simulink model "AFDNFSmodelSPA"  (R2017b)
settings: Solver=ode45  StartTime=0.0  StopTime=1400  FixedStep=1e-3  RelTol=1e-8  EnableMultiTasking=on
PostLoadFcn:
  | run('Methods/NFSOnLoad');
InitFcn:
  | run('Methods/AFDSimInit')
StopFcn:
  | run('Methods/NFSOnLoad');
values from neighbouring files (symbols this model uses):
  nfs = TransferFunction('Plot','true')    [Main.m]    (also in NFSDatabase.sldd = SI
                Imperial
                28184.4409185639)
undefined symbols (not defined in the file or in its folder): Continuous, desired, Earth, F, K_lat, K_long, Kobsvlat, Kobsvlong, lat, latsys, Light, long, longsys, MIL, Newton, Raphson, sigbuilder_block, Time, WGS84
libraries: simulink x6, aerolibtransform2 x2, aerolibwind2 x2, ModelsLibrary x1, ctrlSharedLib x1, sharedutil x1
(part 1 of 4)
settings Model: Creator=AHKh PC  LastModifiedBy=AHKh
settings SolverCC: ZeroCrossAlgorithm=Adaptive  AutoInsertRateTranBlk=on
settings DataIOCC: SaveFormat=Array  SignalLoggingSaveFormat=ModelDataLogs  SaveOutput=off
settings OptimizationCC: ExpressionDepthLimit=2147483647  LifeSpan=inf
settings DebuggingCC: UnderspecifiedInitializationDetection=Classic  MergeDetectMultiDrivingBlocksExec=none  SolverPrmCheckMsg=warning  FcnCallInpInsideContextMsg=warning  StateNameClashWarn=warning  SFUnexpectedBacktrackingDiag=warning  SFNoUnconditionalDefaultTransitionDiag=warning  SFExecutionAtInitializationDiag=none
settings HardwareCC: ProdBitPerPointer=32  ProdBitPerSizeT=32  ProdBitPerPtrDiffT=32  ProdLargestAtomicFloat=None  ProdIntDivRoundTo=Undefined  ProdEndianess=Unspecified  ProdWordSize=32  ProdHWDeviceType=32-bit Generic
settings ModelReferenceCC: PropagateSignalLabelsOutOfModel=off
settings CodeAppCC: StateflowObjectComments=on
settings GRTTargetCC: TargetLangStandard=C89/C90 (ANSI)  GeneratePreprocessorConditionals=Disable all
settings ConfigComp: CovMetricSettings=dw  CovHtmlReporting=on  CovSaveCumulativeToWorkspaceVar=on  CovSaveSingleToWorkspaceVar=on  CovExternalEMLEnable=off

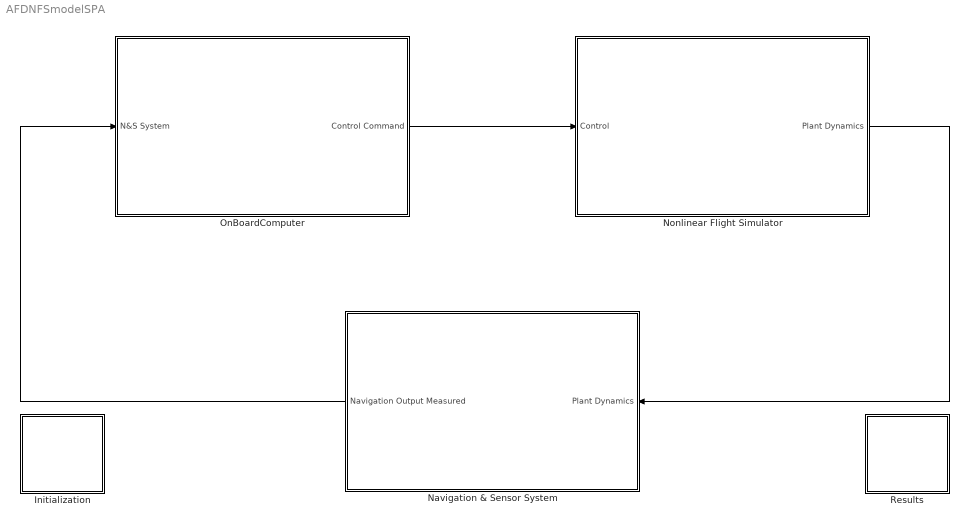
== system AFDNFSmodelSPA ==
  Initialization : Subsystem
      settings: OpenFcn=|
      | % edit('Methods/AFDSimInit.m')
      | !NFSData/NFS Data.xlsx
      mask Display: image(imread('iData/Initialization'))
  Navigation & Sensor System : Subsystem
      mask Display: image(imread('iData/NavigationSystem'))
  Nonlinear Flight Simulator : Subsystem
      mask Display: image(imread('iData/LockheedMartinVARIOUS'));
  OnBoardComputer : Subsystem
      mask Display: image(imread('iData/OnBoardComputerESAPathfinder'));
  Results : Subsystem
      settings: OpenFcn=|
      | cd 'Methods';
      | Plotter(ned_position,euler_angles,control_commands,tout)
      | cd ..
      mask Display: image(imread('iData/Initialization'))
  wires:
  OnBoardComputer/1(Control Command) -> Nonlinear Flight Simulator/1(Control)
  Navigation & Sensor System/1(Navigation Output Measured) -> OnBoardComputer/1(N&S System)
  Nonlinear Flight Simulator/1(Plant Dynamics) -> Navigation & Sensor System/1(Plant Dynamics)

== system AFDNFSmodelSPA/Initialization ==

== system AFDNFSmodelSPA/Navigation & Sensor System ==
  note: Major Contributions
      | 1- Pitotube Model Shall be added
      | 2- GPS Model shall be added
      | 3-
      | 4-
  note: 0-Ideal Measurement - full-state feedback
      |
      | 1- Test Model - no filter propagation - model based propagation
      |
      | 2- Pure noise added to all measurements - no filter - full-state feedback
      |
      | 3- Pure noise added to all measurements - Linear Kalman Filter - gyro and accelerometer feedback - postion ideal
      |
      | 4- Pure noise added to all measurements - Extended Kalman Filter - gyro and accelerometer feedback - postion ideal
      |
      | 5- Pure noise added to all measurements - Unscented Kalman Filter - gyro and accelerometer feedback - postion ideal
      |
      | 6 - Comprehensive model of Gyro and Accelerometer - Extended Kalman Filter - Ideal Position
      |
      | 7 - Comprehensive model of Gyro and Accelerometer - Unscented Kalman Filter - Ideal Position
      |
      | 8 - Adding GPS to equations
  Plant Dynamics : Inport
  Navigation Model : Subsystem  Variant=on
  Navigation Output Measured : Outport
  wires:
  Plant Dynamics/1 -> Navigation Model/1(In)
  Navigation Model/1(Out) -> Navigation Output Measured/1

== system AFDNFSmodelSPA/Nonlinear Flight Simulator ==
  Control : Inport
  6DoF Nonlinear Flight Equations of Motion (Rigid Body) : Subsystem
  Bus Creator : BusCreator  Inputs=7
  Forces and Moments : Subsystem
  Ground1 : Ground
  Initialization : Subsystem
  Plot : Subsystem
  Scope : Scope
  Scope1 : Scope
  Scope4 : Scope
  Plant Dynamics : Outport
  wires:
  Forces and Moments/1(Force (Body)) -> Scope1/1, 6DoF Nonlinear Flight Equations of Motion (Rigid Body)/1(Forces (F) (Body))
  Forces and Moments/2(Moment (Body)) -> Scope4/1, 6DoF Nonlinear Flight Equations of Motion (Rigid Body)/2(Moments (M) (Body))
  6DoF Nonlinear Flight Equations of Motion (Rigid Body)/1(Linear Velocity (Body)) -> Forces and Moments/1(Linear Velocity), Bus Creator/1, Plot/1(Linear Velocity (Body))  "Linear Velocity"
  Initialization/3(Initial Inertia tensor) -> 6DoF Nonlinear Flight Equations of Motion (Rigid Body)/5(Inertia Tensor (I))
  Initialization/4(Inertia tensor Change Rate) -> 6DoF Nonlinear Flight Equations of Motion (Rigid Body)/6(Inertia Tensor Change Rate (Idot))
  Control/1 -> Forces and Moments/3(Control)
  Initialization/2(Mass Consumption Rate) -> 6DoF Nonlinear Flight Equations of Motion (Rigid Body)/4(Mass Consumption Rate)
  Initialization/1(Initial Mass) -> 6DoF Nonlinear Flight Equations of Motion (Rigid Body)/3(Initial Mass)
  Initialization/5(Initial Linear Velocity Vector) -> 6DoF Nonlinear Flight Equations of Motion (Rigid Body)/7(Initial Linear Velocity Vector)
  Initialization/6(Initial Angular Velocity Vector) -> 6DoF Nonlinear Flight Equations of Motion (Rigid Body)/8(Initial Angular Velocity Vector)
  Initialization/7(Initial Euler Angles) -> 6DoF Nonlinear Flight Equations of Motion (Rigid Body)/9(Initial Euler Angles)
  6DoF Nonlinear Flight Equations of Motion (Rigid Body)/2(Angular Velocity (Body)) -> Forces and Moments/2(Angular Velocity), Bus Creator/2, Plot/2(Angular Velocity (Body))  "Angular Velocity"
  6DoF Nonlinear Flight Equations of Motion (Rigid Body)/4(Angular Acceleration (Body)) -> Bus Creator/4, Plot/4(Angular Acceleration (Body))  "Angular Acceleration"
  Initialization/8(Initial Location (NED)) -> 6DoF Nonlinear Flight Equations of Motion (Rigid Body)/10(Initial Location (NED))
  6DoF Nonlinear Flight Equations of Motion (Rigid Body)/3(Linear Acceleration (Body)) -> Bus Creator/3, Plot/3(Linear Acceleration (Body))  "Linear Acceleration"
  6DoF Nonlinear Flight Equations of Motion (Rigid Body)/7(Velocity (NED)) -> Bus Creator/7, Plot/7(Velocity (NED))  "Velocity"
  Ground1/1 -> Scope/1
  6DoF Nonlinear Flight Equations of Motion (Rigid Body)/6(Position (NED)) -> Forces and Moments/5(Position), Bus Creator/6, Plot/6(Position (NED))  "Position"
  6DoF Nonlinear Flight Equations of Motion (Rigid Body)/5(Euler Angles) -> Forces and Moments/4(Attitute), Bus Creator/5, Plot/5(Euler Angles)  "Euler Angles"
  Bus Creator/1 -> Plant Dynamics/1
  6DoF Nonlinear Flight Equations of Motion (Rigid Body)/8(T_BI) -> Forces and Moments/6(T_BI)

== system AFDNFSmodelSPA/OnBoardComputer ==
  N&S System : Inport
  Control System : Subsystem
  Guidance Algorithm : Subsystem
  Control Command : Outport
  wires:
  N&S System/1 -> Control System/2(N&S System), Guidance Algorithm/1(N&S System)
  Guidance Algorithm/1(Guidance Command) -> Control System/1(Guidance)
  Control System/1(Control Command) -> Control Command/1

== system AFDNFSmodelSPA/Results ==

== system AFDNFSmodelSPA/Navigation & Sensor System/Navigation Model ==
  In : Inport
  00-Ideal Measurement : Subsystem  VariantControl=NavigationSelector == 0
  01-Test Model : Subsystem  VariantControl=NavigationSelector == 1
  02-Pure Noise Full-State Feedback : Subsystem  VariantControl=NavigationSelector == 2
  03-Pure Noise Linear Kalman Filter (LKF) : Subsystem  VariantControl=NavigationSelector == 3
  Out : Outport

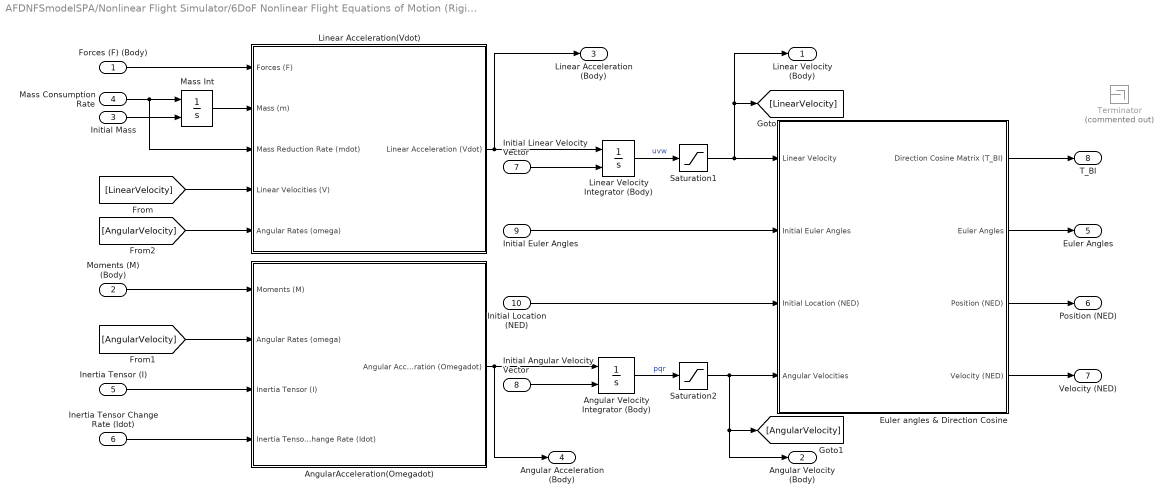
== system AFDNFSmodelSPA/Nonlinear Flight Simulator/6DoF Nonlinear Flight Equations of Motion (Rigid Body) ==
  Forces (F) (Body) : Inport
  Moments (M) (Body) : Inport  Port=2  PortDimensions=[3,1]
  Initial Mass : Inport  Port=3
  Mass Consumption Rate : Inport  Port=4
  Inertia Tensor (I) : Inport  Port=5
  Inertia Tensor Change Rate (Idot) : Inport  Port=6
  Initial Linear Velocity Vector : Inport  Port=7
  Initial Angular Velocity Vector : Inport  Port=8
  Initial Euler Angles : Inport  Port=9
  Initial Location (NED) : Inport  Port=10
  Angular Velocity Integrator (Body) : Integrator  InitialConditionSource=external  InitialCondition=nfs.angularvel0
  AngularAcceleration(Omegadot) : Subsystem
  Euler angles & Direction Cosine : Subsystem
  Linear Acceleration(Vdot) : Subsystem
  Linear Velocity Integrator (Body) : Integrator  InitialConditionSource=external  InitialCondition=nfs.crusevelvec  ContinuousStateAttributes='BodyVelocity'
  Mass Int : Integrator  InitialConditionSource=external  InitialCondition=nfs.crusevelvec  ContinuousStateAttributes='BodyVelocity'
  Saturation1 : Saturate  UpperLimit=500  LowerLimit=-500
  Saturation2 : Saturate  UpperLimit=500  LowerLimit=-500
  Terminator : Terminator  Commented=on
  Linear Velocity (Body) : Outport
  Angular Velocity (Body) : Outport  Port=2
  Linear Acceleration (Body) : Outport  Port=3
  Angular Acceleration (Body) : Outport  Port=4
  Euler Angles : Outport  Port=5
  Position (NED) : Outport  Port=6
  Velocity (NED) : Outport  Port=7
  T_BI : Outport  Port=8
  wires:
  Initial Mass/1 -> Mass Int/2
  Mass Int/1 -> Linear Acceleration(Vdot)/2(Mass (m))
  Mass Consumption Rate/1 -> Linear Acceleration(Vdot)/3(Mass Reduction Rate (mdot)), Mass Int/1
  Linear Velocity Integrator (Body)/1 -> Saturation1/1  "uvw"
  Angular Velocity Integrator (Body)/1 -> Saturation2/1  "pqr"
  Inertia Tensor (I)/1 -> AngularAcceleration(Omegadot)/3(Inertia Tensor (I))
  Inertia Tensor Change Rate (Idot)/1 -> AngularAcceleration(Omegadot)/4(Inertia Tensor Change Rate (Idot))
  Euler angles & Direction Cosine/1(Direction Cosine Matrix (T_BI)) -> T_BI/1
  Initial Location (NED)/1 -> Euler angles & Direction Cosine/3(Initial Location (NED))
  Forces (F) (Body)/1 -> Linear Acceleration(Vdot)/1(Forces (F))
  Linear Acceleration(Vdot)/1(Linear Acceleration (Vdot)) -> Linear Acceleration (Body)/1, Linear Velocity Integrator (Body)/1
  Initial Linear Velocity Vector/1 -> Linear Velocity Integrator (Body)/2
  Initial Angular Velocity Vector/1 -> Angular Velocity Integrator (Body)/2
  AngularAcceleration(Omegadot)/1(Angular Acceleration (Omegadot)) -> Angular Velocity Integrator (Body)/1, Angular Acceleration (Body)/1
  [LinearVelocity] -> Linear Acceleration(Vdot)/4(Linear Velocities (V))
  [AngularVelocity] -> Linear Acceleration(Vdot)/5(Angular Rates (omega))
  Moments (M) (Body)/1 -> AngularAcceleration(Omegadot)/1(Moments (M))
  [AngularVelocity] -> AngularAcceleration(Omegadot)/2(Angular Rates (omega))
  Initial Euler Angles/1 -> Euler angles & Direction Cosine/2(Initial Euler Angles)
  Euler angles & Direction Cosine/4(Velocity (NED)) -> Velocity (NED)/1
  Euler angles & Direction Cosine/2(Euler Angles) -> Euler Angles/1
  Euler angles & Direction Cosine/3(Position (NED)) -> Position (NED)/1
  Saturation1/1 -> Linear Velocity (Body)/1, [LinearVelocity], Euler angles & Direction Cosine/1(Linear Velocity)
  Saturation2/1 -> Angular Velocity (Body)/1, [AngularVelocity], Euler angles & Direction Cosine/4(Angular Velocities)

== system AFDNFSmodelSPA/Nonlinear Flight Simulator/Forces and Moments ==
  Linear Velocity : Inport
  Angular Velocity : Inport  Port=2
  Control : Inport  Port=3
  Attitute : Inport  Port=4  PortDimensions=[3,1]
  Position : Inport  Port=5
  T_BI : Inport  Port=6
  "Aerodynamic Forces and " : Subsystem
  Constant : Constant  Value=[0;0;9.806]
  From : From  Commented=on  GotoTag=Gravity
  Goto1 : Goto  Commented=on  GotoTag=Gravity
  Gravity Calculator : Subsystem
  Sum{,1..3} (4 alike) : Sum  Inputs=|++
  Thrust : Subsystem
  Weight : Subsystem
  Force (Body) : Outport
  Moment (Body) : Outport  Port=2
  wires:
  [Altitude] -> "Aerodynamic Forces and "/5(Altitude)
  Attitute/1 -> Weight/1(Attitute)
  Position/1 -> Gravity Calculator/1(Position (NED))
  Gravity Calculator/2(Altitud) -> [Altitude]
  Sum2/1 -> Force (Body)/1
  Linear Velocity/1 -> "Aerodynamic Forces and "/1(Linear Velocity)
  T_BI/1 -> "Aerodynamic Forces and "/4(T_BI)
  Weight/1(Weight Force) -> Sum2/2
  "Aerodynamic Forces and "/2(Moment (Body)) -> Sum1/1
  Sum1/1 -> Sum3/1
  Gravity Calculator/1(Gravity (NED)) -> Goto1/1
  Thrust/2(Thrust Moment) -> Sum1/2
  "Aerodynamic Forces and "/1(Force (Body)) -> Sum/1
  Sum/1 -> Sum2/1
  Control/1 -> "Aerodynamic Forces and "/3(Control)
  Weight/2(Weight Moment) -> Sum3/2
  Sum3/1 -> Moment (Body)/1
  Angular Velocity/1 -> "Aerodynamic Forces and "/2(Angular Velocity 1)
  Thrust/1(Thrust Force) -> Sum/2
  Constant/1 -> Weight/2(Gravity)

== system AFDNFSmodelSPA/Nonlinear Flight Simulator/Initialization ==
  Constant : Constant  Value=nfs.mass
  Constant1 : Constant  Value=nfs.consumprate
  Constant2 : Constant  Value=nfs.I
  Constant3 : Constant  Value=zeros(3)
  Constant4 : Constant  Value=nfs.crusevelvec
  Constant6 : Constant  Value=nfs.angularvel0
  Constant7 : Constant  Value=nfs.attitude0
  Constant8 : Constant  Value=nfs.initialpos
  Reshape1 : Reshape
  Reshape2 : Reshape  OutputDimensionality=Customize  OutputDimensions=[3,3]
  Reshape3 : Reshape  OutputDimensionality=Customize  OutputDimensions=[3,3]
  Reshape{4,6..8} (4 alike) : Reshape  OutputDimensionality=Column vector (2-D)
  Reshape5 : Reshape
  Initial Mass : Outport
  Mass Consumption Rate : Outport  Port=2
  Initial Inertia tensor : Outport  Port=3
  Inertia tensor Change Rate : Outport  Port=4
  Initial Linear Velocity Vector : Outport  Port=5
  Initial Angular Velocity Vector : Outport  Port=6
  Initial Euler Angles : Outport  Port=7
  Initial Location (NED) : Outport  Port=8
  wires:
  Constant/1 -> Reshape5/1
  Constant1/1 -> Reshape1/1
  Constant2/1 -> Reshape2/1
  Constant3/1 -> Reshape3/1
  Constant4/1 -> Reshape4/1
  Constant6/1 -> Reshape6/1
  Constant7/1 -> Reshape7/1
  Constant8/1 -> Reshape8/1
  Reshape5/1 -> Initial Mass/1
  Reshape1/1 -> Mass Consumption Rate/1
  Reshape2/1 -> Initial Inertia tensor/1
  Reshape3/1 -> Inertia tensor Change Rate/1
  Reshape4/1 -> Initial Linear Velocity Vector/1
  Reshape6/1 -> Initial Angular Velocity Vector/1
  Reshape7/1 -> Initial Euler Angles/1
  Reshape8/1 -> Initial Location (NED)/1

== system AFDNFSmodelSPA/Nonlinear Flight Simulator/Plot ==
  Linear Velocity (Body) : Inport
  Angular Velocity (Body) : Inport  Port=2
  Linear Acceleration (Body) : Inport  Port=3
  Angular Acceleration (Body) : Inport  Port=4
  Euler Angles : Inport  Port=5  PortDimensions=3
  Position (NED) : Inport  Port=6  PortDimensions=3
  Velocity (NED) : Inport  Port=7
  Angular Acceleration - (Body) : Scope
  Angular Velocity - (Body) : Scope
  Cockpit Monitors : Subsystem  Commented=on
  Euler Angles1 : Scope
  Euler Angles2 : InportShadow  Port=5  PortDimensions=3
  Gain{,1..2,5} (4 alike) : Gain  Gain=180/pi
  Gain3 : Gain  Gain=[1,1,-1]'
  Gain4 : Gain  Gain=[1,1,-1]'
  Linear Acceleration - (Body) : Scope
  Linear Velocity - (Body) : Scope
  Position (NED)1 : InportShadow  Port=6  PortDimensions=3
  Position - (NED) : Scope
  To Workspace : ToWorkspace  VariableName=ned_position  SampleTime=-1
  To Workspace1 : ToWorkspace  VariableName=euler_angles  SampleTime=-1
  Velocity - (NED) : Scope
  wires:
  Gain/1 -> Euler Angles1/1
  Euler Angles/1 -> Gain/1
  Position (NED)/1 -> Gain3/1
  Linear Velocity (Body)/1 -> Linear Velocity - (Body)/1
  Angular Velocity (Body)/1 -> Gain2/1
  Linear Acceleration (Body)/1 -> Linear Acceleration - (Body)/1
  Angular Acceleration (Body)/1 -> Gain1/1
  Velocity (NED)/1 -> Velocity - (NED)/1
  Gain1/1 -> Angular Acceleration - (Body)/1
  Gain2/1 -> Angular Velocity - (Body)/1
  Gain3/1 -> Position - (NED)/1
  Position (NED)1/1 -> Gain4/1
  Gain4/1 -> To Workspace/1
  Euler Angles2/1 -> Gain5/1
  Gain5/1 -> To Workspace1/1

== system AFDNFSmodelSPA/OnBoardComputer/Control System ==
  Guidance : Inport
  N&S System : Inport  Port=2
  Constant2 : Constant  Value=[0 0 0 0]'
  Demux : Demux
  Ground2 : Ground  Commented=on
  LQR : Subsystem  SystemSampleTime=1
      settings: MinAlgLoopOccurrences=on
  Manual Switch1 : ManualSwitch  CurrentSetting=0
  Mux : Mux
  Scope : Scope
  Sum : Sum  Inputs=++|
  Terminator{,1..3} (4 alike) : Terminator  Commented=on
  Terminator4 : Terminator
  To Workspace1 : ToWorkspace  VariableName=control_commands  SampleTime=-1
  Trim Offset + Reference Excitation : Subsystem
  Unfinished Controllers (State-Feedback) : Subsystem  Commented=on
  Control Command : Outport
  wires:
  Sum/1 -> Scope/1, Control Command/1, To Workspace1/1
  [delta_e] -> Mux/1
  [delta_f] -> Mux/2
  [delta_a] -> Mux/3
  [delta_r] -> Mux/4
  Trim Offset + Reference Excitation/1(Trim) -> Sum/1
  Mux/1 -> Manual Switch1/1
  Constant2/1 -> Manual Switch1/2
  Manual Switch1/1 -> Sum/2
  Ground2/1 -> Unfinished Controllers (State-Feedback)/1(Reference Input)
  Unfinished Controllers (State-Feedback)/1(dE) -> Terminator/1
  Unfinished Controllers (State-Feedback)/2(dF) -> Terminator1/1
  Unfinished Controllers (State-Feedback)/3(dA) -> Terminator2/1
  Unfinished Controllers (State-Feedback)/4(dR) -> Terminator3/1
  Guidance/1 -> Terminator4/1
  N&S System/1 -> LQR/1(N&S System)
  Demux/1 -> [delta_e]
  Demux/2 -> [delta_f]
  Demux/3 -> [delta_a]
  Demux/4 -> [delta_r]
  LQR/1(Control Command) -> Demux/1

== system AFDNFSmodelSPA/OnBoardComputer/Guidance Algorithm ==
  N&S System : Inport
  Bus Creator{,5..6,8} (4 alike) : BusCreator  Inputs=2
  Bus Creator1 : BusCreator  Inputs=1
  Bus Creator2 : BusCreator  Inputs=1
  Bus Creator3 : BusCreator  Inputs=3
  Bus Creator4 : BusCreator  Inputs=1
  Bus Creator7 : BusCreator  Inputs=3
  Bus Selector : BusSelector  OutputSignals=Linear Velocity,Angular Velocity,Linear Acceleration,Angular Acceleration,Euler Angles,Position,Velocity
  Constant : Constant  Value=desired.pitch
  Constant1 : Constant  Value=[nfs.crusevelvec(1); nfs.crusevelvec(3)]
  Constant2 : Constant  Value=nfs.crusevelvec(2)
  Demux : Demux  Outputs=2
  Demux1 : Demux  Outputs=2
  Demux2 : Demux  Outputs=2
  Selector : Selector  InputPortWidth=3  IndexOptions=Index vector (dialog)  Indices=[2]  OutputSizes=1
  Selector1 : Selector  InputPortWidth=3  IndexOptions=Index vector (dialog)  Indices=[2]  OutputSizes=1
  Selector2 : Selector  InputPortWidth=3  IndexOptions=Index vector (dialog)  Indices=[2]  OutputSizes=1
  Selector3 : Selector  InputPortWidth=3  IndexOptions=Index vector (dialog)  Indices=[1 3]  OutputSizes=1
  Selector4 : Selector  InputPortWidth=3  IndexOptions=Index vector (dialog)  Indices=[1 3]  OutputSizes=1
  Selector5 : Selector  InputPortWidth=3  IndexOptions=Index vector (dialog)  Indices=[1 3]  OutputSizes=1
  Sum : Sum  Inputs=|+-
  Sum1 : Sum  Inputs=-+|
  Sum2 : Sum  Inputs=|+-
  Terminator{1..4} (4 alike) : Terminator
  Guidance Command : Outport
  wires:
  N&S System/1 -> Bus Selector/1
  Bus Selector/1 -> Selector3/1, Selector1/1  "<Linear Velocity>"
  Bus Selector/3 -> Terminator1/1  "<Linear Acceleration>"
  Bus Selector/4 -> Terminator2/1  "<Angular Acceleration>"
  Bus Selector/7 -> Terminator4/1  "<Velocity>"
  Bus Selector/2 -> Selector/1, Selector4/1  "<Angular Velocity>"
  Bus Selector/6 -> Terminator3/1  "<Position>"
  Bus Selector/5 -> Selector2/1, Selector5/1  "<Euler Angles>"
  Selector/1 -> Bus Creator1/1  "q_error"
  Selector4/1 -> Demux1/1  "p & r"
  Selector5/1 -> Demux2/1  "phi & psi"
  Selector2/1 -> Sum/1  "Theta"
  Sum/1 -> Bus Creator2/1  "theta_error"
  Constant/1 -> Sum/2
  Sum1/1 -> Demux/1
  Selector3/1 -> Sum1/2  "u & w"
  Constant1/1 -> Sum1/1
  Selector1/1 -> Sum2/1  "v"
  Sum2/1 -> Bus Creator4/1  "v_error"
  Constant2/1 -> Sum2/2
  Demux/1 -> Bus Creator/1  "u_error"
  Demux/2 -> Bus Creator/2  "w_error"
  Bus Creator/1 -> Bus Creator3/1  "Linear Velocity Error"
  Bus Creator1/1 -> Bus Creator3/2  "Angular Rate Error"
  Bus Creator2/1 -> Bus Creator3/3  "Angular Error"
  Demux1/2 -> Bus Creator5/2  "r_error"
  Demux1/1 -> Bus Creator5/1  "p_error"
  Demux2/1 -> Bus Creator6/1  "phi_error"
  Demux2/2 -> Bus Creator6/2  "psi_error"
  Bus Creator4/1 -> Bus Creator7/1  "Linear Velocity Error"
  Bus Creator5/1 -> Bus Creator7/2  "Angular Rate Error"
  Bus Creator6/1 -> Bus Creator7/3  "Angular Error"
  Bus Creator8/1 -> Guidance Command/1
  Bus Creator3/1 -> Bus Creator8/1  "Longitudinal Reference Error"
  Bus Creator7/1 -> Bus Creator8/2  "Lateral-Directional Reference Error"

== system AFDNFSmodelSPA/Navigation & Sensor System/Navigation Model/00-Ideal Measurement ==
  In : Inport
  Out : Outport
  wires:
  In/1 -> Out/1

== system AFDNFSmodelSPA/Navigation & Sensor System/Navigation Model/01-Test Model ==
  In : Inport
  3Axis IMU - Measurement Model : ModelsLibrary/3Axis IMU  units=Metric (MKS)  IMULocation=nfs.Measurement.IMULoc  Ts=nfs.Measurement.Rate  AccSubtractGravity=off  dtype_a=on  AccNaturalFrequency=190  AccDampingRatio=0.707  AccSFCC=nfs.Measurement.Acc.SFCC  AccMeasurmentBias=[0; 0; 0]  AccMeasUpperLimit=[inf; inf; inf]  AccMeasLowerLimit=[-inf; -inf; -inf]  AccNoiseCheck=on  AccNoiseSeeds=nfs.Measurement.Acc.Seed  AccNoisePower=nfs.Measurement.Acc.NoisePower  dtype_g=on  GyroNaturalFrequency=190  GyroDampingRatio=0.707  GyroSFCC=nfs.Measurement.Gyro.SFCC  GyroMeasurmentBias=[0; 0; 0]  GyroGSensitiveBias=[0; 0; 0]  GyroMeasUpperLimit=[inf; inf; inf]  GyroMeasLowerLimit=[-inf; -inf; -inf]  GyroNoiseCheck=on  GyroNoiseSeeds=nfs.Measurement.Gyro.Seed  GyroNoisePower=nfs.Measurement.Gyro.NoisePower
  Bus Creator : BusCreator  Inputs=7
  Bus Selector : BusSelector  OutputSignals=Linear Velocity,Angular Velocity,Linear Acceleration,Angular Acceleration,Euler Angles,Position,Velocity
  CG Loc in Body : Constant  Value=[0;0;0]
  Gravity Calculator : Subsystem
  Initialization : Subsystem
  Navigation Model - Simple : Subsystem
  Product : Product  Multiplication=Matrix(*)
  Terminator{1,4..6} (4 alike) : Terminator
  Out : Outport
  wires:
  In/1 -> Bus Selector/1
  Gravity Calculator/1(Gravity (NED)) -> Product/2
  Navigation Model - Simple/3(Euler Angles Measured) -> Bus Creator/5  "Euler Angles"
  Navigation Model - Simple/4(Position (NED) Measured) -> Bus Creator/6, Gravity Calculator/1(Position (NED))  "Position"
  Bus Selector/3 -> 3Axis IMU - Measurement Model/1  "<Linear Acceleration>"
  Bus Creator/1 -> Out/1
  Navigation Model - Simple/6(T_BI Measured) -> Product/1
  Bus Selector/7 -> Terminator4/1  "<Velocity>"
  Bus Selector/4 -> 3Axis IMU - Measurement Model/3  "<Angular Acceleration>"
  Navigation Model - Simple/1(Linear Velocity (Body) Measured) -> Bus Creator/1  "Linear Velocity"
  Navigation Model - Simple/5(Velocity (NED) Measured) -> Bus Creator/7  "Velocity"
  Initialization/3(Initial Euler Angles) -> Navigation Model - Simple/5(Initial Euler Angles)
  Initialization/2(Initial Angular Velocity Vector) -> Navigation Model - Simple/4(Initial Angular Velocity Vector)
  CG Loc in Body/1 -> 3Axis IMU - Measurement Model/4
  Bus Selector/5 -> Terminator5/1  "<Euler Angles>"
  Initialization/4(Initial Location (NED)) -> Navigation Model - Simple/6(Initial Location (NED))
  Initialization/1(Initial Linear Velocity Vector) -> Navigation Model - Simple/3(Initial Linear Velocity Vector)
  Product/1 -> 3Axis IMU - Measurement Model/5
  Bus Selector/1 -> Terminator6/1  "<Linear Velocity>"
  Bus Selector/6 -> Terminator1/1  "<Position>"
  Bus Selector/2 -> 3Axis IMU - Measurement Model/2  "<Angular Velocity>"
  3Axis IMU - Measurement Model/1 -> Bus Creator/3, Navigation Model - Simple/1(Linear Acceleration (Body))  "Linear Acceleration"
  Navigation Model - Simple/2(Angular Velocity (Body) Measured) -> Bus Creator/2  "Angular Velocity"
  3Axis IMU - Measurement Model/2 -> Bus Creator/4, Navigation Model - Simple/2(Angular Acceleration (Body))  "Angular Acceleration"

== system AFDNFSmodelSPA/Navigation & Sensor System/Navigation Model/02-Pure Noise Full-State Feedback ==
  In : Inport
  Band-Limited White Noise : simulink/Sources/Band-Limited White Noise  Cov=nfs.Uncertainty.Noise.Power  Ts=nfs.Uncertainty.Noise.SampleTime  seed=[630548]
  Band-Limited White Noise1 : simulink/Sources/Band-Limited White Noise  Cov=nfs.Uncertainty.Noise.Power  Ts=nfs.Uncertainty.Noise.SampleTime  seed=[630548]
  Band-Limited White Noise2 : simulink/Sources/Band-Limited White Noise  Cov=nfs.Uncertainty.Noise.Power  Ts=nfs.Uncertainty.Noise.SampleTime  seed=[630548]
  Bus Creator : BusCreator  Inputs=7
  Bus Selector : BusSelector  OutputSignals=Linear Velocity,Angular Velocity,Linear Acceleration,Angular Acceleration,Euler Angles,Position,Velocity
  Sum : Sum  Inputs=++|
  Sum1 : Sum  Inputs=++|
  Sum2 : Sum  Inputs=++|
  Out : Outport
  wires:
  In/1 -> Bus Selector/1
  Bus Selector/3 -> Bus Creator/3  "<Linear Acceleration>"
  Bus Selector/4 -> Bus Creator/4  "<Angular Acceleration>"
  Bus Selector/6 -> Bus Creator/6  "<Position>"
  Bus Selector/7 -> Bus Creator/7  "<Velocity>"
  Bus Selector/1 -> Sum/2  "<Linear Velocity>"
  Band-Limited White Noise/1 -> Sum/1
  Bus Selector/2 -> Sum1/2  "<Angular Velocity>"
  Band-Limited White Noise1/1 -> Sum1/1
  Bus Selector/5 -> Sum2/2  "<Euler Angles>"
  Band-Limited White Noise2/1 -> Sum2/1
  Sum/1 -> Bus Creator/1  "Linear Velocity"
  Sum1/1 -> Bus Creator/2  "Angular Velocity"
  Sum2/1 -> Bus Creator/5  "Euler Angles"
  Bus Creator/1 -> Out/1

== system AFDNFSmodelSPA/Navigation & Sensor System/Navigation Model/03-Pure Noise Linear Kalman Filter (LKF) ==
  In : Inport
  Band-Limited White Noise : simulink/Sources/Band-Limited White Noise  Cov=nfs.Uncertainty.Noise.Power  Ts=nfs.Uncertainty.Noise.SampleTime  seed=[630548]
  Band-Limited White Noise1 : simulink/Sources/Band-Limited White Noise  Cov=nfs.Uncertainty.Noise.Power  Ts=nfs.Uncertainty.Noise.SampleTime  seed=[630548]
  Band-Limited White Noise2 : simulink/Sources/Band-Limited White Noise  Cov=nfs.Uncertainty.Noise.Power  Ts=nfs.Uncertainty.Noise.SampleTime  seed=[630548]
  Bus Creator : BusCreator  Inputs=7
  Bus Selector : BusSelector  OutputSignals=Linear Velocity,Angular Velocity,Linear Acceleration,Angular Acceleration,Euler Angles,Position,Velocity
  Kalman Filter : ctrlSharedLib/Kalman Filter  TimeDomain=Continuous-Time  UseCurrentEstimator=on  ModelSource=Individual A, B, C, D matrices  ModelSourceVariable=ss(0.95,1,1,0,1)  A=nfs.dyn.linsys.A  B=1  C=nfs.dyn.linsys.C  D=0  NumberOfStates=1  NumberOfInputs=1  NumberOfOutputs=1  InitialEstimateSource=Dialog  X0=0  P0=10  UseK=off  UseGH=off  NumberOfProcessNoiseInputs=1  G=1  TimeInvariantG=on  H=0  TimeInvariantH=on  Q=eye(9)  TimeInvariantQ=on  R=eye(9)  TimeInvariantR=on  N=zeros(size(nfs.dyn.linsys.A))  TimeInvariantN=on  AddInputPort=off  AddEnablePort=off  OutputEstimatedY=off  OutputP=off  Ts=-1
      settings: SourceProductBaseCode=CT
  Mux : Mux  Inputs=3
  Mux1 : Mux  Inputs=3
  Mux2 : Mux  Inputs=2
  Selector : Selector  InputPortWidth=3  IndexOptions=Index vector (dialog)  Indices=[1 3]  OutputSizes=1
  Selector1 : Selector  InputPortWidth=3  IndexOptions=Index vector (dialog)  Indices=[2]  OutputSizes=1
  Selector2 : Selector  InputPortWidth=3  IndexOptions=Index vector (dialog)  Indices=[2]  OutputSizes=1
  Selector3 : Selector  InputPortWidth=3  IndexOptions=Index vector (dialog)  Indices=[2]  OutputSizes=1
  Selector4 : Selector  InputPortWidth=3  IndexOptions=Index vector (dialog)  Indices=[1 3]  OutputSizes=1
  Selector5 : Selector  InputPortWidth=3  IndexOptions=Index vector (dialog)  Indices=[1 3]  OutputSizes=1
  Selector6 : Selector  InputPortWidth=9  IndexOptions=Index vector (dialog)  Indices=[1 5 2 6 3 7 8 4 9]  OutputSizes=1
  Selector7 : Selector  InputPortWidth=9  IndexOptions=Index vector (dialog)  Indices=[1 2 3]  OutputSizes=1
  Selector8 : Selector  InputPortWidth=9  IndexOptions=Index vector (dialog)  Indices=[4 5 6]  OutputSizes=1
  Selector9 : Selector  InputPortWidth=9  IndexOptions=Index vector (dialog)  Indices=[7 8 9]  OutputSizes=1
  Sum : Sum  Inputs=++|
  Sum1 : Sum  Inputs=++|
  Sum2 : Sum  Inputs=++|
  Out : Outport
  wires:
  Bus Creator/1 -> Out/1
  Sum2/1 -> Selector2/1  "Euler Angles"
  Sum1/1 -> Selector1/1, Selector4/1, Selector5/1  "Angular Velocity"
  Sum/1 -> Selector/1, Selector3/1  "Linear Velocity"
  Band-Limited White Noise2/1 -> Sum2/1
  Bus Selector/5 -> Sum2/2  "<Euler Angles>"
  Band-Limited White Noise1/1 -> Sum1/1
  Bus Selector/2 -> Sum1/2  "<Angular Velocity>"
  Band-Limited White Noise/1 -> Sum/1
  Bus Selector/1 -> Sum/2  "<Linear Velocity>"
  Bus Selector/7 -> Bus Creator/7  "<Velocity>"
  Bus Selector/6 -> Bus Creator/6  "<Position>"
  Bus Selector/4 -> Bus Creator/4  "<Angular Acceleration>"
  Bus Selector/3 -> Bus Creator/3  "<Linear Acceleration>"
  In/1 -> Bus Selector/1
  Selector/1 -> Mux/1
  Selector1/1 -> Mux/2
  Selector2/1 -> Mux/3
  Selector3/1 -> Mux1/1
  Selector4/1 -> Mux1/2
  Selector5/1 -> Mux1/3
  Mux1/1 -> Mux2/2
  Mux/1 -> Mux2/1
  Mux2/1 -> Kalman Filter/1
  Kalman Filter/1 -> Selector6/1
  Selector6/1 -> Selector9/1, Selector7/1, Selector8/1
  Selector7/1 -> Bus Creator/1  "Linear Velocity"
  Selector8/1 -> Bus Creator/2  "Angular Velocity"
  Selector9/1 -> Bus Creator/5  "Euler Angles"

== system AFDNFSmodelSPA/Nonlinear Flight Simulator/6DoF Nonlinear Flight Equations of Motion (Rigid Body)/AngularAcceleration(Omegadot) ==
  Moments (M) : Inport  PortDimensions=[3,1]
  Angular Rates (omega) : Inport  Port=2  PortDimensions=[3,1]
  Inertia Tensor (I) : Inport  Port=3
  Inertia Tensor Change Rate (Idot) : Inport  Port=4
  Angular Rates (omega)1 : InportShadow  Port=2  PortDimensions=[3,1]
  Cross Product : Subsystem  mask(Cross Product){}
      mask help: Calculate the cross product of two 3-by-1 vectors.
      mask Display:
      | text(.5,.5,'Cross\nProduct\nC = AxB', ...
      | 	'HorizontalAlignment','Center',...
      | 	'VerticalAlignment','middle')
  Inertia Tensor (I)1 : InportShadow  Port=3
  Product1 : Product  Inputs=**  Multiplication=Matrix(*)  SaturateOnIntegerOverflow=on  OutDataTypeStr=Inherit: Same as first input
  Product3 : Product  Inputs=**  Multiplication=Matrix(*)  SaturateOnIntegerOverflow=on  OutDataTypeStr=Inherit: Same as first input
  Product4 : Product  Inputs=/*  Multiplication=Matrix(*)  SaturateOnIntegerOverflow=on  OutDataTypeStr=Inherit: Same as first input
  Sum1 : Sum  Inputs=|+-  SaturateOnIntegerOverflow=on
  Sum3 : Sum  Inputs=|+-  SaturateOnIntegerOverflow=on
  Angular Acceleration (Omegadot) : Outport
  wires:
  Product3/1 -> Sum1/2
  Product1/1 -> Cross Product/2(B)
  Cross Product/1(C) -> Sum3/2
  Sum1/1 -> Sum3/1
  Sum3/1 -> Product4/2
  Product4/1 -> Angular Acceleration (Omegadot)/1
  Inertia Tensor (I)1/1 -> Product4/1
  Moments (M)/1 -> Sum1/1
  Inertia Tensor Change Rate (Idot)/1 -> Product3/1
  Angular Rates (omega)/1 -> Cross Product/1(A), Product3/2
  Angular Rates (omega)1/1 -> Product1/2
  Inertia Tensor (I)/1 -> Product1/1

== system AFDNFSmodelSPA/Nonlinear Flight Simulator/6DoF Nonlinear Flight Equations of Motion (Rigid Body)/Euler angles & Direction Cosine ==
  Linear Velocity : Inport  PortDimensions=[3,1]
  Initial Euler Angles : Inport  Port=2
  Initial Location (NED) : Inport  Port=3  PortDimensions=[3,1]
  Angular Velocities : Inport  Port=4
  Constant : Constant
  Euler Angles Int : Integrator  InitialConditionSource=external  InitialCondition=nfs.attitude0
  Euler angles Calculation : Subsystem
  If : If  IfExpression=u1(3)>= 0  ShowElse=off
  If Action Subsystem : Subsystem  TreatAsAtomicUnit=on
  Position Integrator : Integrator  InitialConditionSource=external  InitialCondition=[0,0,nfs.attitude0]
  Rotation Angles to DCM : Subsystem
  Selector : Selector  InputPortWidth=3  IndexOptions=Index vector (dialog)  Indices=[3 2 1]  OutputSizes=1
  Transform from Body to Inertial axes : Subsystem
      mask Display: disp('T_IB')
  Transpose : Math  Operator=transpose  SaturateOnIntegerOverflow=on
  Direction Cosine Matrix (T_BI) : Outport  PortDimensions=[3,3]
  Euler Angles : Outport  Port=2
  Position (NED) : Outport  Port=3  PortDimensions=[3,1]
  Velocity (NED) : Outport  Port=4  PortDimensions=[3,1]
  wires:
  Initial Euler Angles/1 -> Euler Angles Int/2
  Rotation Angles to DCM/1(DCM) -> Transpose/1, Direction Cosine Matrix (T_BI)/1
  Angular Velocities/1 -> Euler angles Calculation/1(Angular Velocities)
  Selector/1 -> Rotation Angles to DCM/1("[R1,R2,R3]")
  Transpose/1 -> Transform from Body to Inertial axes/1(Transformation Matrix)
  Linear Velocity/1 -> Transform from Body to Inertial axes/2(Position Vector)
  Initial Location (NED)/1 -> Position Integrator/2
  Euler Angles Int/1 -> Euler Angles/1, Selector/1, Euler angles Calculation/2(Euler Angles)
  Transform from Body to Inertial axes/1(Ve) -> Velocity (NED)/1, Position Integrator/1
  Position Integrator/1 -> Position (NED)/1, If/1
  Euler angles Calculation/1(Euler Rates) -> Euler Angles Int/1
  If/1 -> If Action Subsystem/Action
  Constant/1 -> If Action Subsystem/1(Simulation Termination)

== system AFDNFSmodelSPA/Nonlinear Flight Simulator/6DoF Nonlinear Flight Equations of Motion (Rigid Body)/Linear Acceleration(Vdot) ==
  Forces (F) : Inport  PortDimensions=[3,1]
  Mass (m) : Inport  Port=2
  Mass Reduction Rate (mdot) : Inport  Port=3
  Linear Velocities (V) : Inport  Port=4  PortDimensions=[3,1]
  Angular Rates (omega) : Inport  Port=5
  Cross Product : Subsystem  mask(Cross Product){}
      mask help: Calculate the cross product of two 3-by-1 vectors.
      mask Display:
      | text(.5,.5,'Cross\nProduct\nC = AxB', ...
      | 	'HorizontalAlignment','Center',...
      | 	'VerticalAlignment','middle')
  Linear Velocities (V)1 : InportShadow  Port=4  PortDimensions=[3,1]
  Mass (m)1 : InportShadow  Port=2
  Product : Product  Inputs=*/  SaturateOnIntegerOverflow=on  OutDataTypeStr=Inherit: Same as first input
  Product1 : Product  Inputs=*/  SaturateOnIntegerOverflow=on  OutDataTypeStr=Inherit: Same as first input
  Product3 : Product  Inputs=**  SaturateOnIntegerOverflow=on  OutDataTypeStr=Inherit: Same as first input
  Sum1 : Sum  Inputs=|+-  SaturateOnIntegerOverflow=on
  Sum3 : Sum  Inputs=|+-  SaturateOnIntegerOverflow=on
  Linear Acceleration (Vdot) : Outport
  wires:
  Mass (m)/1 -> Product/2
  Product/1 -> Sum1/1
  Mass Reduction Rate (mdot)/1 -> Product1/1
  Mass (m)1/1 -> Product1/2
  Product1/1 -> Product3/1
  Product3/1 -> Sum1/2
  Sum1/1 -> Sum3/1
  Cross Product/1(C) -> Sum3/2
  Linear Velocities (V)/1 -> Product3/2
  Forces (F)/1 -> Product/1
  Sum3/1 -> Linear Acceleration (Vdot)/1
  Angular Rates (omega)/1 -> Cross Product/1(A)
  Linear Velocities (V)1/1 -> Cross Product/2(B)

== system AFDNFSmodelSPA/Nonlinear Flight Simulator/Forces and Moments/Aerodynamic Forces and  ==
  Linear Velocity : Inport
  Angular Velocity 1 : Inport  Port=2
  Control : Inport  Port=3
  T_BI : Inport  Port=4
  Altitude : Inport  Port=5
  Aero Attributes : Subsystem
  Angular Velocity : InportShadow  Port=2
  Bus Selector : BusSelector  OutputSignals=Linear Velocity,Angular Velocity
  Control1 : InportShadow  Port=3
  Energy Analysis1 : Subsystem  Commented=on  mask{ae=nfs}
      mask prompts: ae "Aero Coefficients"
  Forces : Subsystem
  From : From  Commented=on  GotoTag=alpha
  From1 : From  Commented=on  GotoTag=beta
  From2 : From  Commented=on  GotoTag=betadot
  From3 : From  Commented=on  GotoTag=alphadot
  From4 : From  Commented=on  GotoTag=DynPress
  Goto : Goto  Commented=on  GotoTag=alpha
  Goto1 : Goto  Commented=on  GotoTag=beta
  Goto2 : Goto  Commented=on  GotoTag=betadot
  Goto3 : Goto  Commented=on  GotoTag=alphadot
  Goto4 : Goto  Commented=on  GotoTag=DynPress
  Linear Velocity1 : InportShadow
  Moments : Subsystem
  Scope{,1..5} (6 alike) : Scope  Commented=on
  Turbulence : Subsystem
  Force (Body) : Outport
  Moment (Body) : Outport  Port=2
  wires:
  Angular Velocity 1/1 -> Energy Analysis1/4(Angular Vel Body)
  Energy Analysis1/1(Lift) -> Scope/1
  From3/1 -> Energy Analysis1/6(Alpha_dot)
  Bus Selector/1 -> Forces/1(Linear Velocity), Moments/1(Linear Velocity), Aero Attributes/1(Linear Velocity (Body))  "<Linear Velocity>"
  Energy Analysis1/6(Z Moment) -> Scope5/1
  T_BI/1 -> Turbulence/4(DCM)
  Altitude/1 -> Turbulence/3(Altitude), Aero Attributes/2(Altitude)
  Moments/1(Aerodynamic Moments (Body)) -> Moment (Body)/1
  Energy Analysis1/3(Y Moment) -> Scope2/1
  Forces/1(Aerodynamic Forces (Body)) -> Force (Body)/1
  Aero Attributes/5(Betadot) -> Goto2/1
  Linear Velocity/1 -> Turbulence/1(Linear Velocity)
  From1/1 -> Energy Analysis1/7(Beta)
  From2/1 -> Energy Analysis1/8(Beta_dot)
  Aero Attributes/6(Mach) -> Forces/8(Mach), Moments/8(Mach)
  Control/1 -> Forces/5(Control), Moments/5(Control)
  Energy Analysis1/2(Drag) -> Scope1/1
  Aero Attributes/2(Beta) -> Goto1/1, Forces/3(Beta), Moments/3(Beta)
  Aero Attributes/4(Alphadot) -> Goto3/1, Forces/7(Alphadot), Moments/7(Alphadot)
  From4/1 -> Energy Analysis1/1(Dynamic Pressure)
  Energy Analysis1/4(Side Force) -> Scope3/1
  Energy Analysis1/5(X Moment) -> Scope4/1
  Aero Attributes/1(Alpha) -> Goto/1, Forces/2(Alpha), Moments/2(Alpha)
  Linear Velocity1/1 -> Energy Analysis1/3(Linear Vel Body)
  From/1 -> Energy Analysis1/5(Alpha)
  Control1/1 -> Energy Analysis1/2(Control)
  Aero Attributes/3(Dynamic Pressure) -> Goto4/1, Forces/6(Dynamic Pressure), Moments/6(Dynamic Pressure)
  Bus Selector/2 -> Forces/4(Angular Velocity), Moments/4(Angular Velocity)  "<Angular Velocity>"
  Angular Velocity/1 -> Turbulence/2(Angular Velocity)
  Turbulence/1(Turbulent Velocity) -> Bus Selector/1

== system AFDNFSmodelSPA/Nonlinear Flight Simulator/Forces and Moments/Gravity Calculator ==
  Position (NED) : Inport
  Flat Earth to LLA : aerolibtransform2/Flat Earth to LLA  units=Metric (MKS)  ptype=Earth (WGS84)  F=1/298.257223563  R=6378137  LL0=[nfs.Coordinate.Lat nfs.Coordinate.Long]  psi=0
  Mux1 : Mux  Inputs=2
  Ref Alt : Constant  Value=0
  Reshape : Reshape  OutputDimensionality=Customize  OutputDimensions=[1,3]
  Reshape1 : Reshape  OutputDimensionality=Customize  OutputDimensions=[3,1]
  "WGS84 Gravity Model  " : GravityWGS84
  Gravity (NED) : Outport
  Altitud : Outport  Port=2
  wires:
  Mux1/1 -> Reshape/1
  Flat Earth to LLA/2 -> Mux1/2, Altitud/1
  Reshape/1 -> "WGS84 Gravity Model  "/1
  Flat Earth to LLA/1 -> Mux1/1
  Position (NED)/1 -> Flat Earth to LLA/1
  Ref Alt/1 -> Flat Earth to LLA/2
  "WGS84 Gravity Model  "/1 -> Reshape1/1
  Reshape1/1 -> Gravity (NED)/1

== system AFDNFSmodelSPA/Nonlinear Flight Simulator/Forces and Moments/Thrust ==
  Manual Switch : ManualSwitch  CurrentSetting=0
  Mux1 : Mux  Inputs=3
  Product : Product  RndMeth=Zero
  Signal Builder : Subsystem  Tag=STV Subsys  LoadFcn=sigbuilder_block('load');  StartFcn=sigbuilder_block('start');  StopFcn=sigbuilder_block('stop');  ClipboardFcn=sigbuilder_block('clipboard');  mask(Sigbuilder block){tuvar=[0:10]}
      mask help: Simulink:masks:SigbuilderBlock_MD
      mask init:
      | if ~strcmp(get_param(bdroot(gcbh),'SimulationStatus'),'stopped') tuvar = sigbuilder_block('maskInit'); end
      settings: CopyFcn=sigbuilder_block('copy');  DeleteFcn=sigbuilder_block('delete');  ModelCloseFcn=sigbuilder_block('modelClose');  PreSaveFcn=sigbuilder_block('preSave');  PauseFcn=sigbuilder_block('pause');  ContinueFcn=sigbuilder_block('continue');  NameChangeFcn=sigbuilder_block('namechange');  OpenFcn=sigbuilder_block('open',[437.25 199.5 550.5 399.75 ]);  CloseFcn=sigbuilder_block('close');
      mask Display: plot(0, 0, 100, 100,[2, 2, 32, 32, 2], [68, 8, 8, 68, 68],[32, 2], [38, 38], [32, 19, 2],[53, 60, 44], [32, 17, 17, 2],[16, 16, 31, 31]);txt = getActiveGroup(gcbh);text(2, 100, txt,'verticalAlignment', 'top');
  Throttle : Gain
  Trim Thrust1 : Constant  Value=nfs.trim.thrust*cos(nfs.tmisalign)
  Trim Thrust2 : Constant  Value=nfs.trim.thrust*sin(nfs.tmisalign)
  Trim Thrust3 : Constant  Value=0
  Trim Thrust4 : Constant
  Trim Thrust5 : Constant  Value=[0;0;0]
  Thrust Force : Outport  PortDimensions=[3,1]
  Thrust Moment : Outport  Port=2  PortDimensions=[3,1]
  wires:
  Mux1/1 -> Throttle/1
  Trim Thrust3/1 -> Mux1/3
  Trim Thrust2/1 -> Mux1/2
  Trim Thrust1/1 -> Mux1/1
  Throttle/1 -> Product/1
  Product/1 -> Thrust Force/1
  Manual Switch/1 -> Product/2
  Signal Builder/1(ThrustDeviation) -> Manual Switch/1
  Trim Thrust4/1 -> Manual Switch/2
  Trim Thrust5/1 -> Thrust Moment/1

== system AFDNFSmodelSPA/Nonlinear Flight Simulator/Forces and Moments/Weight ==
  note: theta
  note: phi
  Attitute : Inport  PortDimensions=[3,1]
  Gravity : Inport  Port=2  PortDimensions=[3,1]
  Demux : Demux  Outputs=3
  Gain1 : Gain  Gain=-1
  Mux1 : Mux  Inputs=3
  Product{1..2,4..5} (4 alike) : Product  RndMeth=Zero
  Terminator4 : Terminator
  Trigonometric Function1 : Trigonometry  Operator=cos
  Trigonometric Function2 : Trigonometry
  Trigonometric Function3 : Trigonometry  Operator=cos
  Trigonometric Function4 : Trigonometry
  Trim Thrust5 : Constant  Value=[0;0;0]
  Vector Magnitude : Subsystem
  mass : Constant  Value=nfs.mass
  Weight Force : Outport  PortDimensions=[3,1]
  Weight Moment : Outport  Port=2  PortDimensions=[3,1]
  wires:
  Mux1/1 -> Product2/1
  Product5/1 -> Mux1/3
  Product4/1 -> Mux1/2
  Gain1/1 -> Mux1/1
  Trigonometric Function1/1 -> Product5/2
  Trigonometric Function4/1 -> Product4/1
  Trigonometric Function3/1 -> Product5/1, Product4/2
  Trigonometric Function2/1 -> Gain1/1
  mass/1 -> Product1/1
  Demux/3 -> Terminator4/1
  Attitute/1 -> Demux/1
  Demux/2 -> Trigonometric Function3/1, Trigonometric Function2/1
  Demux/1 -> Trigonometric Function1/1, Trigonometric Function4/1
  Trim Thrust5/1 -> Weight Moment/1
  Gravity/1 -> Vector Magnitude/1(Vector)
  Product1/1 -> Product2/2
  Product2/1 -> Weight Force/1
  Vector Magnitude/1(Vector Magnitude) -> Product1/2

== system AFDNFSmodelSPA/Nonlinear Flight Simulator/Plot/Cockpit Monitors ==
  Airspeed Indicator : Subsystem  DialogController=aeroblksHMICreateDDGDialog  IsWebBlock=on  mask(MWDashboardBlock){webBlockId=212af7a9-24bf-41a0-9308-db922aa4261c, webBlockType=airspeedindicator, ShowInLibBrowser=on, ShowInitialText=on, HMISrcModelName=AFDNFSmodelSPA}
      mask prompts: webBlockId "WebBlock Id"; webBlockType "WebBlock Type"; HMISrcModelName "Source Model"
      mask help: aeroblksHMI:aeroblkhmi:AirspeedIndicatorDialogDesc
      mask Help: eval('asbhmihelp(''airspeedindicator'')');
      mask Display:
      | if strcmp(get_param(bdroot(gcb),'BlockDiagramType'), 'library')
      |  image([(matlabroot) '/toolbox/aeroblks/aeroblks/hmi/icons/AirspeedIndicatorIcon.svg'])
      | end

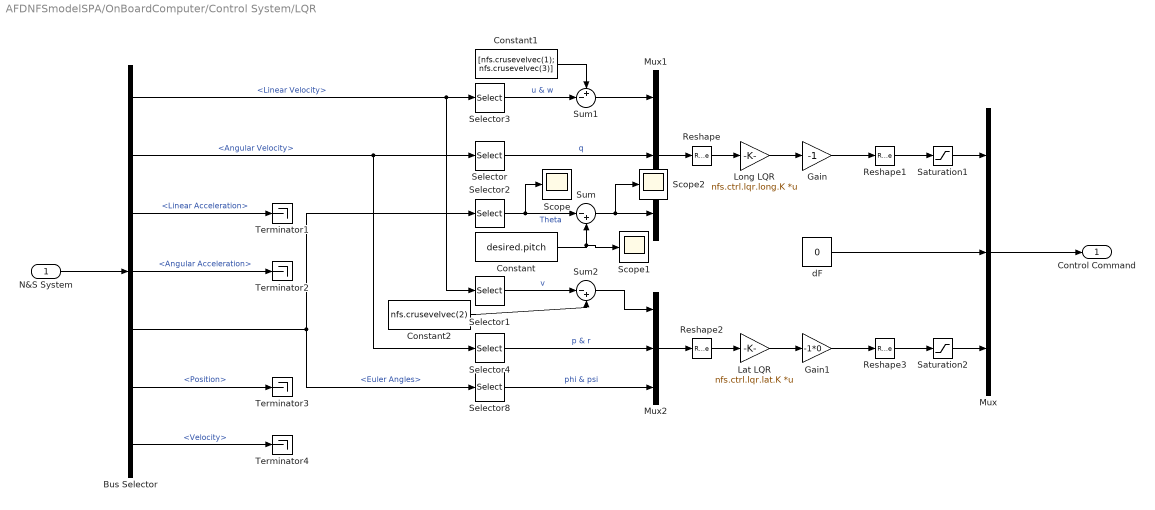
== system AFDNFSmodelSPA/OnBoardComputer/Control System/LQR ==
  N&S System : Inport
  Bus Selector : BusSelector  OutputSignals=Linear Velocity,Angular Velocity,Linear Acceleration,Angular Acceleration,Euler Angles,Position,Velocity
  Constant : Constant  Value=desired.pitch
  Constant1 : Constant  Value=[nfs.crusevelvec(1); nfs.crusevelvec(3)]
  Constant2 : Constant  Value=nfs.crusevelvec(2)
  Gain : Gain  Gain=-1
  Gain1 : Gain  Gain=-1*0
  Lat LQR : Gain  Gain=nfs.ctrl.lqr.lat.K  Multiplication=Matrix(K*u)
  Long LQR : Gain  Gain=nfs.ctrl.lqr.long.K  Multiplication=Matrix(K*u)
  Mux : Mux  Inputs=3
  Mux1 : Mux  Inputs=3
  Mux2 : Mux  Inputs=3
  Reshape : Reshape  OutputDimensionality=Customize  OutputDimensions=[4,1]
  Reshape1 : Reshape  OutputDimensionality=Customize
  Reshape2 : Reshape  OutputDimensionality=Customize  OutputDimensions=[5,1]
  Reshape3 : Reshape  OutputDimensionality=Customize  OutputDimensions=[2,1]
  Saturation1 : Saturate  UpperLimit=deg2rad(20)  LowerLimit=-deg2rad(20)
  Saturation2 : Saturate  UpperLimit=deg2rad(20)  LowerLimit=-deg2rad(20)
  Scope : Scope
  Scope1 : Scope
  Scope2 : Scope
  Selector : Selector  InputPortWidth=3  IndexOptions=Index vector (dialog)  Indices=[2]  OutputSizes=1
  Selector1 : Selector  InputPortWidth=3  IndexOptions=Index vector (dialog)  Indices=[2]  OutputSizes=1
  Selector2 : Selector  InputPortWidth=3  IndexOptions=Index vector (dialog)  Indices=[2]  OutputSizes=1
  Selector3 : Selector  InputPortWidth=3  IndexOptions=Index vector (dialog)  Indices=[1 3]  OutputSizes=1
  Selector4 : Selector  InputPortWidth=3  IndexOptions=Index vector (dialog)  Indices=[1 3]  OutputSizes=1
  Selector8 : Selector  InputPortWidth=3  IndexOptions=Index vector (dialog)  Indices=[1 3]  OutputSizes=1
  Sum : Sum  Inputs=|-+
  Sum1 : Sum  Inputs=+-|
  Sum2 : Sum  Inputs=|-+
  Terminator{1..4} (4 alike) : Terminator
  dF : Constant  Value=0
  Control Command : Outport
  wires:
  Constant1/1 -> Sum1/1
  Constant2/1 -> Sum2/2
  Sum2/1 -> Mux2/1
  Selector1/1 -> Sum2/1  "v"
  Bus Selector/4 -> Terminator2/1  "<Angular Acceleration>"
  Selector/1 -> Mux1/2  "q"
  Selector4/1 -> Mux2/2  "p & r"
  Bus Selector/1 -> Selector3/1, Selector1/1  "<Linear Velocity>"
  Constant/1 -> Scope1/1, Sum/2
  Bus Selector/2 -> Selector/1, Selector4/1  "<Angular Velocity>"
  Bus Selector/6 -> Terminator3/1  "<Position>"
  Sum1/1 -> Mux1/1
  Bus Selector/7 -> Terminator4/1  "<Velocity>"
  Bus Selector/5 -> Selector8/1, Selector2/1  "<Euler Angles>"
  Sum/1 -> Scope2/1, Mux1/3
  Bus Selector/3 -> Terminator1/1  "<Linear Acceleration>"
  Selector3/1 -> Sum1/2  "u & w"
  Selector2/1 -> Scope/1, Sum/1  "Theta"
  N&S System/1 -> Bus Selector/1
  Mux1/1 -> Reshape/1
  Long LQR/1 -> Gain/1
  Lat LQR/1 -> Gain1/1
  Mux2/1 -> Reshape2/1
  dF/1 -> Mux/2
  Mux/1 -> Control Command/1
  Reshape/1 -> Long LQR/1
  Reshape1/1 -> Saturation1/1
  Reshape2/1 -> Lat LQR/1
  Gain/1 -> Reshape1/1
  Reshape3/1 -> Saturation2/1
  Gain1/1 -> Reshape3/1
  Selector8/1 -> Mux2/3  "phi & psi"
  Saturation1/1 -> Mux/1
  Saturation2/1 -> Mux/3

== system AFDNFSmodelSPA/OnBoardComputer/Control System/Trim Offset + Reference Excitation ==
  Controlled Plant : Constant  Value=[0;0;0;0]
  Doublet Generated Signal : Subsystem
  Free Plant : Constant  Value=[nfs.trim.delta_e+.06;0;0;0]
  Manual Switch : ManualSwitch  CurrentSetting=0
  Manual Switch1 : ManualSwitch  CurrentSetting=0
  Manual Switch2 : ManualSwitch
  Triangular signal span 10 sec : Subsystem
  Trim : Outport
  wires:
  Free Plant/1 -> Manual Switch/2
  Doublet Generated Signal/1(Doublet Out) -> Manual Switch1/1
  Triangular signal span 10 sec/1(Tri) -> Manual Switch1/2
  Manual Switch1/1 -> Manual Switch/1
  Manual Switch/1 -> Manual Switch2/1
  Controlled Plant/1 -> Manual Switch2/2
  Manual Switch2/1 -> Trim/1

== system AFDNFSmodelSPA/OnBoardComputer/Control System/Unfinished Controllers (State-Feedback) ==
  Reference Input : Inport
  Demux : Demux  Outputs=2
  Demux1 : Demux  Outputs=2
  Full-State Feedback Servo : Subsystem
  Full-State Observer Servo : Subsystem
  Ground : Ground
  Ground1 : Ground
  Ground2 : Ground
  Manual Switch{2,4..6} (4 alike) : ManualSwitch  CurrentSetting=0
  Manual Switch3 : ManualSwitch
  Reduced Order Observer Servo : Subsystem
  Scope : Scope
  Scope1 : Scope
  Terminator : Terminator
  Terminator1 : Terminator
  dE : Outport
  dF : Outport  Port=2
  dA : Outport  Port=3
  dR : Outport  Port=4
  wires:
  Reduced Order Observer Servo/1(Longitudinal Control) -> Terminator/1
  Reduced Order Observer Servo/2(Lateral-Directional Control) -> Terminator1/1
  Full-State Observer Servo/2(Lateral-Directional Control) -> Manual Switch5/2
  Full-State Feedback Servo/1(Longitudinal Control) -> Scope/1, Manual Switch4/1
  Ground1/1 -> Manual Switch3/2
  Ground/1 -> Manual Switch2/2
  Demux/1 -> dE/1
  [U] -> Full-State Observer Servo/2(U)
  Manual Switch5/1 -> Demux1/1
  Manual Switch4/1 -> Demux/1
  Full-State Feedback Servo/2(Lateral-Directional Control) -> Manual Switch5/1
  Demux1/2 -> dR/1
  Reference Input/1 -> Scope1/1, Manual Switch3/1, Manual Switch6/1, Manual Switch2/1
  Manual Switch2/1 -> Full-State Observer Servo/1(States)
  Demux1/1 -> dA/1
  Manual Switch3/1 -> Full-State Feedback Servo/1(States)
  Demux/2 -> dF/1
  Manual Switch6/1 -> Reduced Order Observer Servo/1(States)
  Ground2/1 -> Manual Switch6/2
  Full-State Observer Servo/1(Longitudinal Control) -> Manual Switch4/2

== system AFDNFSmodelSPA/Navigation & Sensor System/Navigation Model/01-Test Model/Gravity Calculator ==
  Position (NED) : Inport
  Flat Earth to LLA : aerolibtransform2/Flat Earth to LLA  units=Metric (MKS)  ptype=Earth (WGS84)  F=1/298.257223563  R=6378137  LL0=[nfs.Coordinate.Lat nfs.Coordinate.Long]  psi=0
  Mux1 : Mux  Inputs=2
  Ref Alt : Constant  Value=0
  Reshape : Reshape  OutputDimensionality=Customize  OutputDimensions=[1,3]
  Reshape1 : Reshape  OutputDimensionality=Customize  OutputDimensions=[3,1]
  "WGS84 Gravity Model  " : GravityWGS84
  Gravity (NED) : Outport
  wires:
  Mux1/1 -> Reshape/1
  Flat Earth to LLA/2 -> Mux1/2
  Reshape/1 -> "WGS84 Gravity Model  "/1
  Flat Earth to LLA/1 -> Mux1/1
  Position (NED)/1 -> Flat Earth to LLA/1
  Ref Alt/1 -> Flat Earth to LLA/2
  "WGS84 Gravity Model  "/1 -> Reshape1/1
  Reshape1/1 -> Gravity (NED)/1
